simulink model "Aufgabe4"  (R2016a)
settings: Solver=FixedStepDiscrete  StartTime=0.0  StopTime=20  RelTol=1e-3
undefined symbols (not defined in the file): gcbh, magnitude, N, rcfiltgaincompat, Tbit5_0
libraries: commdigbbndam3 x2, commrandsrc2 x1, commsink2 x1, NoiseLib_2019 x1, commfilt2 x1, Rectfilter_2012 x1, dspstat3 x1
CloseFcn:
  | rtwprivate ssgencode ModelCloseRequest V2_2ASKbp_wcos_EF
settings Model: Creator=Praktikum  LastModifiedBy=Bornitz
settings DataIOCC: LimitDataPoints=on  SaveFormat=Array
settings OptimizationCC: ExpressionDepthLimit=2147483647  InitFltsAndDblsToZero=on
settings DebuggingCC: SaveWithParameterizedLinksMsg=none  SolverPrmCheckMsg=warning  MultiTaskDSMMsg=warning  MultiTaskCondExecSysMsg=none  StateNameClashWarn=warning  StrictBusMsg=ErrorOnBusTreatedAsVector
settings HardwareCC: ProdBitPerPointer=32  ProdLargestAtomicFloat=None  ProdIntDivRoundTo=Undefined  ProdEndianess=Unspecified  ProdWordSize=32  ProdHWDeviceType=32-bit Generic
settings ModelReferenceCC: PropagateSignalLabelsOutOfModel=off
settings GRTTargetCC: TargetFcnLib=ansi_tfl_tmw.mat  CombineOutputUpdateFcns=off  GRTInterface=on
settings ConfigComp: CovModelRefEnable=Off

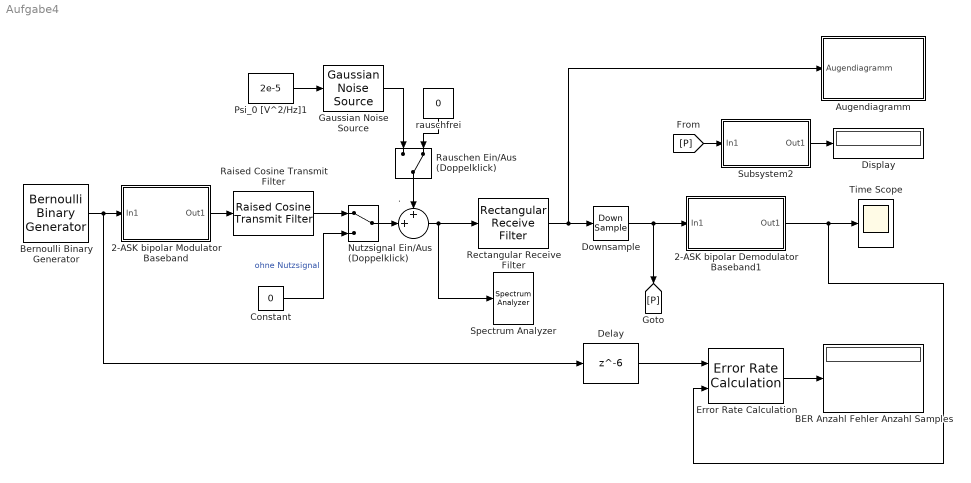
== system Aufgabe4 ==
  . : Sum  Inputs=++|  SampleTime=Tbit5_0/16
  2-ASK bipolar Demodulator Baseband1 : Subsystem
      mask Display:
      | plot(0,0,100,100,[20+1.5*[[0:.8:10] [10:1.6:20] [20:.8:30]] 65 65 65 65+10*[0 1 1 2 2 3]],[85+10*[sin([0:.8:10]*pi*2/5) sin([10:1.6:20]*pi/5) sin([20:.8:30]*pi*2/5)] 85 99 75 85+8*[1 1 -1 -1 1 1]]);
      | disp('\nGeneral\nASK-Demodulator')
  2-ASK bipolar Modulator Baseband : Subsystem
      mask Display:
      | plot(0,0,100,100,[5+15*[0 1 1 2 2 3] 50 50 50 50+1.5*[[0:.8:10] [10:1.6:20] [20:.8:30]]],[85+8*[1 1 -1 -1 1 1] 85 99 75 85+10*[sin([0:.8:10]*pi*2/5) sin([10:1.6:20]*pi/5) sin([20:.8:30]*pi*2/5)]]);
      | disp('\nGeneral\nASK-Modulator')
  Augendiagramm : Subsystem
  BER Anzahl Fehler Anzahl Samples : Display
      settings: Format=short_e
  Bernoulli Binary Generator : commrandsrc2/Bernoulli Binary Generator  P=0.5  seed=61  Ts=Tbit5_0  frameBased=off  sampPerFrame=1  orient=off  outDataType=double
  Constant : Constant  Value=0
  Delay : Delay  DelayLength=6  InitialCondition=0
  Display : Display
  Downsample : DownSample  N=N  phase=8  RateOptions=Allow multirate processing
  Error Rate Calculation : commsink2/Error Rate Calculation  N=0  st_delay=800  cp_mode=Entire frame  subframe=1  PMode=Port  WsName=ErrorVec  RsMode2=off  stop=off  numErr=100  maxBits=1e6
  Gaussian Noise Source : NoiseLib_2019/Gaussian Noise Source  SystemSampleTime=-1
  Nutzsignal Ein/Aus (Doppelklick) : ManualSwitch
  Psi_0 [V^2/Hz]1 : Constant  Value=2e-5
  Raised Cosine Transmit Filter : commfilt2/Raised Cosine Transmit Filter  filtType=Square root  R=0.5  filtSpan=2*(4)  N=N  filterGain=(sqrt(N))*rcfiltgaincompat(gcbh)  RateOptions=Allow multirate processing  framing=Mute  checkCoeff=off  variableName=rcTxFilt  checkGain=User-specified  sampMode=Mute  saveAsFlag=0  currentFiltSpan=2*(4)  D=4  launchFVT=off  roundingMode=Floor  overflowMode=off  coeffDataTypeStr=Inherit: Same word length as input  coeffMin=[]  coeffMax=[]  coeffLastDataTypeStr=Inherit: Same word length as input  outputDataTypeStr=Inherit: Same as accumulator  outputMin=[]  outputMax=[]  outputLastDataTypeStr=Inherit: Same as accumulator
  Rauschen Ein/Aus (Doppelklick) : ManualSwitch  CurrentSetting=0
  Rectangular Receive Filter : Rectfilter_2012/Rectangular Receive Filter  N=N
  Spectrum Analyzer : SpectrumAnalyzer
  Subsystem2 : Subsystem
      mask Display: disp('Leistungs-\n messung')
  Time Scope : Scope
  rauschfrei : Constant  Value=0
  wires:
  Constant/1 -> Nutzsignal Ein/Aus (Doppelklick)/2  "ohne Nutzsignal"
  Rectangular Receive Filter/1 -> Augendiagramm/1(Augendiagramm), Downsample/1
  Bernoulli Binary Generator/1 -> Delay/1, 2-ASK bipolar Modulator Baseband/1(In1)
  rauschfrei/1 -> Rauschen Ein/Aus (Doppelklick)/2
  Gaussian Noise Source/1 -> Rauschen Ein/Aus (Doppelklick)/1
  Rauschen Ein/Aus (Doppelklick)/1 -> ./1
  Nutzsignal Ein/Aus (Doppelklick)/1 -> ./2
  ./1 -> Spectrum Analyzer/1, Rectangular Receive Filter/1
  Raised Cosine Transmit Filter/1 -> Nutzsignal Ein/Aus (Doppelklick)/1
  Error Rate Calculation/1 -> BER Anzahl Fehler Anzahl Samples/1
  Delay/1 -> Error Rate Calculation/1
  Downsample/1 -> [P], 2-ASK bipolar Demodulator Baseband1/1(In1)
  2-ASK bipolar Modulator Baseband/1(Out1) -> Raised Cosine Transmit Filter/1
  2-ASK bipolar Demodulator Baseband1/1(Out1) -> Time Scope/1, Error Rate Calculation/2
  [P] -> Subsystem2/1(In1)
  Psi_0 [V^2/Hz]1/1 -> Gaussian Noise Source/1
  Subsystem2/1(Out1) -> Display/1

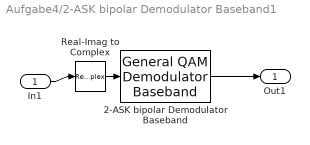
== system Aufgabe4/2-ASK bipolar Demodulator Baseband1 ==
  In1 : Inport
  2-ASK bipolar Demodulator Baseband : commdigbbndam3/General QAM Demodulator Baseband  SigCon=sigdem2  OutType=Bit  DecType=Hard decision  VarSource=Dialog  Variance=1  outDtypeBit=Inherit via internal rule  outDtype=Inherit via internal rule  roundingMode=Floor  overflowMode=Wrap  OvFlMode=off  OvFlModeLastStrValue=off  sigConstWordLen=16  sigConstDataTypeStr=Inherit: Same word length as input  sigConstLastDataTypeStr=Inherit: Same word length as input  accum1WordLen=32  accum1FracLen=30  prodInWordLen=32  prodInFracLen=30  prodInDataTypeStr=Inherit: Same as accumulator 1  prodInLastDataTypeStr=Inherit: Same as accumulator 1  prodOutWordLen=32  prodOutFracLen=30  accum2WordLen=32  accum2FracLen=30  accum3WordLen=32  accum3FracLen=30  nsiWordLen=32  nsiFracLen=30  nsiDataTypeStr=Inherit: Same as accumulator 3  nsiLastDataTypeStr=Inherit: Same as accumulator 3  invn0WordLen=16  invn0FracLen=8  invn0DataTypeStr=Inherit: Same word length as input  invn0LastDataTypeStr=Inherit: Same word length as input  outputWordLen=32  outputFracLen=30
  Real-Imag to Complex : RealImagToComplex  Input=Real
  Out1 : Outport
  wires:
  Real-Imag to Complex/1 -> 2-ASK bipolar Demodulator Baseband/1
  In1/1 -> Real-Imag to Complex/1
  2-ASK bipolar Demodulator Baseband/1 -> Out1/1

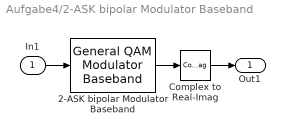
== system Aufgabe4/2-ASK bipolar Modulator Baseband ==
  In1 : Inport
  2-ASK bipolar Modulator Baseband : commdigbbndam3/General QAM Modulator Baseband  SigCon=sig2bp  outDtype=double  outWordLen=16  outUDDataType=sfix(16)  outFracLenMode=Best precision  outFracLen=15  outDataTypeStr=double  outLastDataTypeStr=double
  Complex to Real-Imag : ComplexToRealImag  Output=Real
  Out1 : Outport
  wires:
  2-ASK bipolar Modulator Baseband/1 -> Complex to Real-Imag/1
  In1/1 -> 2-ASK bipolar Modulator Baseband/1
  Complex to Real-Imag/1 -> Out1/1

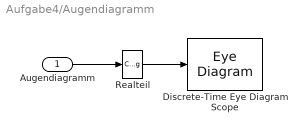
== system Aufgabe4/Augendiagramm ==
  Augendiagramm : Inport
  Discrete-Time Eye Diagram Scope : EyeDiagram  Tag=EyeDiagram
  Realteil : ComplexToRealImag  Output=Real
  wires:
  Augendiagramm/1 -> Realteil/1
  Realteil/1 -> Discrete-Time Eye Diagram Scope/1

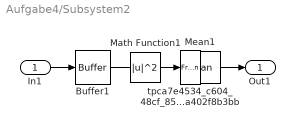
== system Aufgabe4/Subsystem2 ==
  In1 : Inport
  Buffer1 : Buffer  N=5000  TreatMby1Signals=One channel  OutputFrames=off
  Math Function1 : Math  Operator=magnitude^2  SaturateOnIntegerOverflow=on
  Mean1 : dspstat3/Mean  run=off  reset_popup=None  InputProcessing=Columns as channels (frame based)  directionMode=Each column  dimension=1  roiEnable=off  roiType=Rectangles  roiPortion=Entire ROI  roiOutput=Individual statistics for each ROI  roiFlag=off  outputDataTypeStr=Inherit: Same as accumulator  outputLastDataTypeStr=Inherit: Same as accumulator  outputMin=[]  outputMax=[]  roundingMode=Floor  overflowMode=off
  tpca7e4534_c604_48cf_85e7_24a402f8b3bb : FrameConversion  InheritSamplingMode=off
  Out1 : Outport
  wires:
  Math Function1/1 -> Mean1/1
  In1/1 -> Buffer1/1
  Mean1/1 -> Out1/1
  Buffer1/1 -> tpca7e4534_c604_48cf_85e7_24a402f8b3bb/1
  tpca7e4534_c604_48cf_85e7_24a402f8b3bb/1 -> Math Function1/1
